simulink library "mandelbrot_library"  (R2019b)
settings: Solver=VariableStepAuto  StartTime=0.0  StopTime=10.0  RelTol=1e-3
libraries: hdlsllib x2
settings Model: Creator=sasselll  LastModifiedBy=lucas
settings SFSimCC: CustomCodeUndefinedFunction=UseInterfaceOnly

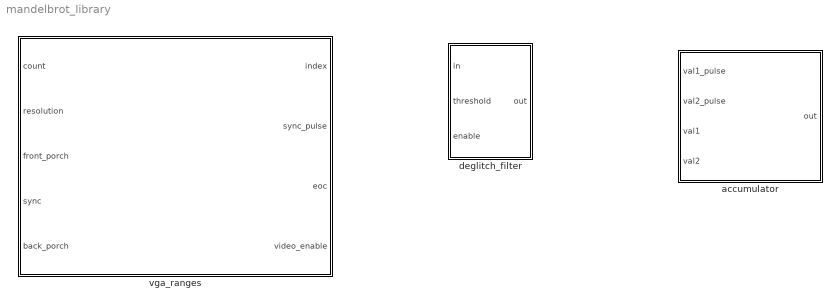
== system mandelbrot_library ==
  accumulator : Subsystem
  deglitch_filter : Subsystem
  vga_ranges : Subsystem

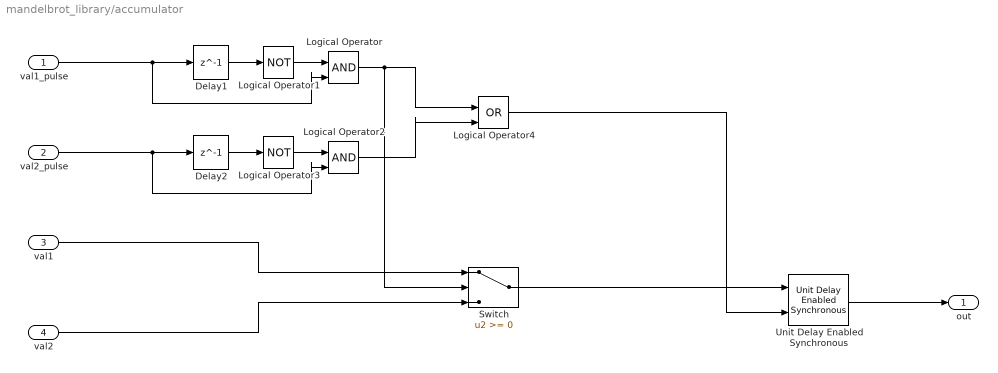
== system mandelbrot_library/accumulator ==
  val1_pulse : Inport
  val2_pulse : Inport  Port=2
  val1 : Inport  Port=3
  val2 : Inport  Port=4
  Delay1 : Delay  DelayLength=1
  Delay2 : Delay  DelayLength=1
  Logical Operator : Logic  IconShape=distinctive  AllPortsSameDT=off  OutDataTypeStr=boolean
  Logical Operator1 : Logic  Operator=NOT  IconShape=distinctive  AllPortsSameDT=off  OutDataTypeStr=boolean
  Logical Operator2 : Logic  IconShape=distinctive  AllPortsSameDT=off  OutDataTypeStr=boolean
  Logical Operator3 : Logic  Operator=NOT  IconShape=distinctive  AllPortsSameDT=off  OutDataTypeStr=boolean
  Logical Operator4 : Logic  Operator=OR  IconShape=distinctive  AllPortsSameDT=off  OutDataTypeStr=boolean
  Switch : Switch
  Unit Delay Enabled Synchronous : hdlsllib/Discrete/Unit Delay Enabled Synchronous  InitialCondition=0.0  SampleTime=-1
      settings: SourceProductName=Simulink  SourceProductBaseCode=SL
  out : Outport  VectorParamsAs1DForOutWhenUnconnected=off
  wires:
  Logical Operator/1 -> Switch/2, Logical Operator4/1
  Delay1/1 -> Logical Operator1/1
  Logical Operator1/1 -> Logical Operator/1
  val1_pulse/1 -> Logical Operator/2, Delay1/1
  val2_pulse/1 -> Logical Operator2/2, Delay2/1
  Logical Operator3/1 -> Logical Operator2/1
  Delay2/1 -> Logical Operator3/1
  Logical Operator2/1 -> Logical Operator4/2
  val1/1 -> Switch/1
  val2/1 -> Switch/3
  Switch/1 -> Unit Delay Enabled Synchronous/1
  Logical Operator4/1 -> Unit Delay Enabled Synchronous/2
  Unit Delay Enabled Synchronous/1 -> out/1

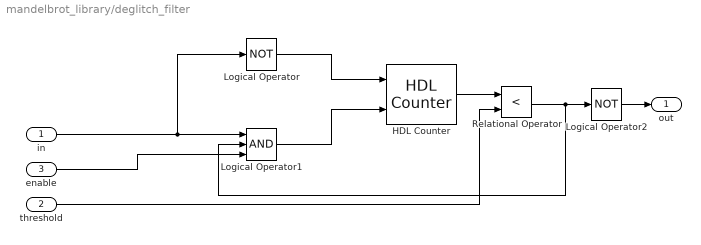
== system mandelbrot_library/deglitch_filter ==
  in : Inport
  threshold : Inport  Port=2
  "enable " : Inport  Port=3
  HDL Counter : hdlsllib/Sources/HDL Counter  CountType=Free running  CountInit=0  CountStep=1  CountMax=25  CountFromType=Initial value  CountFrom=0  CountResetPort=on  CountLoadPort=off  CountEnbPort=on  CountDirPort=off  CountDataType=Unsigned  CountWordLen=8  CountFracLen=0  CountSampTime=1
      settings: SourceProductName=Simulink
  Logical Operator : Logic  Operator=NOT  IconShape=distinctive  AllPortsSameDT=off  OutDataTypeStr=boolean
  Logical Operator1 : Logic  Inputs=3  IconShape=distinctive  AllPortsSameDT=off  OutDataTypeStr=boolean
  Logical Operator2 : Logic  Operator=NOT  IconShape=distinctive  AllPortsSameDT=off  OutDataTypeStr=boolean
  Relational Operator : RelationalOperator  Operator=<  OutDataTypeStr=boolean  RndMeth=Nearest
  out : Outport  VectorParamsAs1DForOutWhenUnconnected=off
  wires:
  Logical Operator1/1 -> HDL Counter/2
  Relational Operator/1 -> Logical Operator2/1, Logical Operator1/2
  threshold/1 -> Relational Operator/2
  in/1 -> Logical Operator1/1, Logical Operator/1
  HDL Counter/1 -> Relational Operator/1
  Logical Operator/1 -> HDL Counter/1
  Logical Operator2/1 -> out/1
  "enable "/1 -> Logical Operator1/3

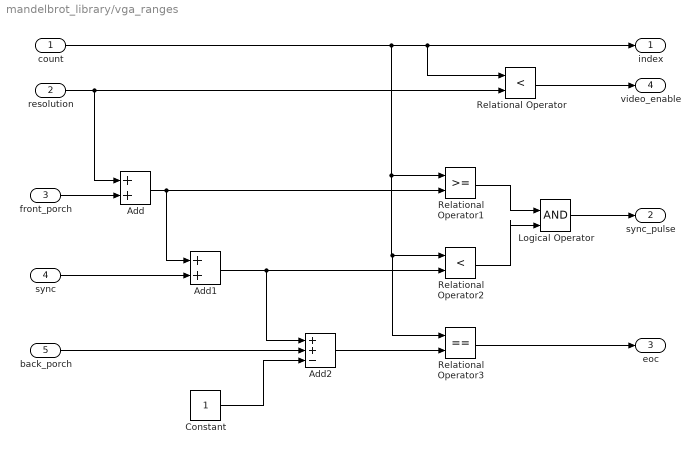
== system mandelbrot_library/vga_ranges ==
  "count " : Inport
  resolution : Inport  Port=2
  front_porch : Inport  Port=3
  "sync " : Inport  Port=4
  back_porch : Inport  Port=5
  Add : Sum
  Add1 : Sum
  Add2 : Sum  Inputs=++-
  Constant : Constant  OutDataTypeStr=Inherit: Inherit via back propagation  SampleTime=-1
  Logical Operator : Logic  IconShape=distinctive  AllPortsSameDT=off  OutDataTypeStr=boolean
  Relational Operator : RelationalOperator  Operator=<  OutDataTypeStr=boolean  RndMeth=Simplest
  Relational Operator1 : RelationalOperator  OutDataTypeStr=boolean  RndMeth=Simplest
  Relational Operator2 : RelationalOperator  Operator=<  OutDataTypeStr=boolean  RndMeth=Simplest
  Relational Operator3 : RelationalOperator  Operator===  OutDataTypeStr=boolean  RndMeth=Simplest
  "index " : Outport
  "sync_pulse " : Outport  Port=2
  "eoc " : Outport  Port=3
  video_enable : Outport  Port=4
  wires:
  resolution/1 -> Add/1, Relational Operator/2
  "count "/1 -> "index "/1, Relational Operator/1, Relational Operator3/1, Relational Operator2/1, Relational Operator1/1
  Relational Operator/1 -> video_enable/1
  front_porch/1 -> Add/2
  "sync "/1 -> Add1/2
  Add/1 -> Add1/1, Relational Operator1/2
  Add1/1 -> Add2/1, Relational Operator2/2
  Relational Operator1/1 -> Logical Operator/1
  Relational Operator2/1 -> Logical Operator/2
  Logical Operator/1 -> "sync_pulse "/1
  back_porch/1 -> Add2/2
  Constant/1 -> Add2/3
  Add2/1 -> Relational Operator3/2
  Relational Operator3/1 -> "eoc "/1
